simulink model "xsens2kinova"  (R2021a)
settings: Solver=FixedStepAuto  StartTime=0.0  StopTime=inf  FixedStep=0.01  RelTol=1e-3
model workspace (MAT data in the model file):
  MAF_len = 80
undefined symbols (not defined in the file): Attitude, Position, VelocityAtt, VelocityPos
libraries: robotlib x7, dspstat3 x6
settings Model: Creator=user  LastModifiedBy=ywchang
settings SolverCC: AlgebraicLoopSolver=TrustRegion
settings OptimizationCC: EnhancedBackFolding=on  PassReuseOutputArgsAs=Individual arguments  ZeroExternalMemoryAtStartup=off  ZeroInternalMemoryAtStartup=off  MaxStackSize=64  OptimizeBlockOrder=speed  DifferentSizesBufferReuse=on  OptimizationCustomize=off  EfficientTunableParamExpr=on
settings DebuggingCC: ParameterTunabilityLossMsg=error  SFMachineParentedDataDiag=warning
settings HardwareCC: ProdBitPerPointer=32  ProdBitPerSizeT=32  ProdBitPerPtrDiffT=32  ProdLargestAtomicFloat=None  ProdIntDivRoundTo=Undefined  ProdEndianess=Unspecified  ProdWordSize=32  ProdHWDeviceType=Generic->Unspecified (assume 32-bit Generic)  UseEmbeddedCoderFeatures=off
settings SFSimCC: MATLABDynamicMemAlloc=off
settings RTWCC: SystemTargetFile=ert.tlc  HardwareBoard=Robot Operating System (ROS)  TLCOptions="-aInlineSetEventsForThisBaseRateFcn=TLC_FALSE -aSuppressMultiTaskScheduler=TLC_FALSE  -aRateBasedStepFcn=0"  TemplateMakefile=ert_default_tmf  Toolchain=Catkin  TargetLang=C++
settings CodeAppCC: ForceParamTrailComments=on  IgnoreCustomStorageClasses=off  OperatorAnnotations=on  SimulinkDataObjDesc=on  SFDataObjDesc=on  InsertBlockDesc=on
settings ERTTargetCC: SupportNonInlinedSFcns=on

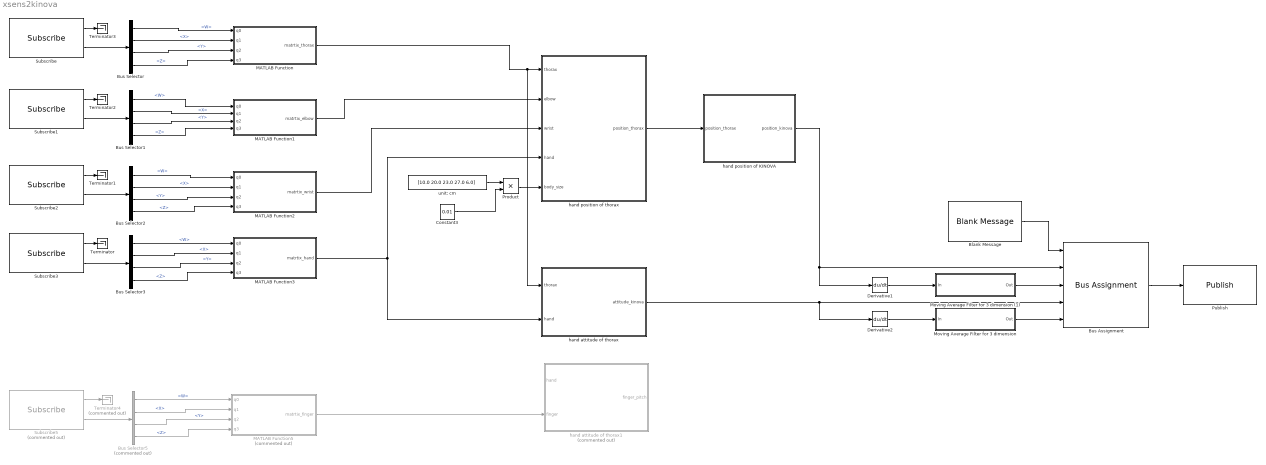
== system xsens2kinova ==
  Blank Message : robotlib/Blank Message  messageClass=Message  entityType=xsens_mtw_driver/xsens2kinova  messageType=xsens_mtw_driver/xsens2kinova  SampleTime=inf  legacyBusStruct=off
  Bus Assignment : BusAssignment  AssignedSignals=Position,VelocityPos,Attitude,VelocityAtt
  Bus Selector{,1..3} (4 alike) : BusSelector  OutputSignals=Orientation.W,Orientation.X,Orientation.Y,Orientation.Z
  Bus Selector5 : BusSelector  Commented=on  OutputSignals=Orientation.W,Orientation.X,Orientation.Y,Orientation.Z
  Constant3 : Constant  Value=0.01
  Derivative1 : Derivative
  Derivative2 : Derivative
  MATLAB Function : MATLAB Function  TreatAsAtomicUnit=on
  MATLAB Function1 : MATLAB Function  TreatAsAtomicUnit=on
  MATLAB Function2 : MATLAB Function  TreatAsAtomicUnit=on
  MATLAB Function3 : MATLAB Function  TreatAsAtomicUnit=on
  MATLAB Function5 : MATLAB Function  Commented=on  TreatAsAtomicUnit=on
  Moving Average Filter for 3 dimension : Subsystem
  Moving Average Filter for 3 dimension (1) : Subsystem
  Product : Product
  Publish : robotlib/Publish  topicSource=Specify your own  topic=/xsens2kinova  messageType=xsens_mtw_driver/xsens2kinova  legacyBusStruct=off  messageQueueLength=1
  Subscribe : robotlib/Subscribe  topicSource=Select from ROS network  topic=/imu_00B47ADF  messageType=sensor_msgs/Imu  SampleTime=-1  legacyBusStruct=off  messageQueueLength=1
  Subscribe1 : robotlib/Subscribe  topicSource=Select from ROS network  topic=/imu_00B47AE4  messageType=sensor_msgs/Imu  SampleTime=-1  legacyBusStruct=off  messageQueueLength=1
  Subscribe2 : robotlib/Subscribe  topicSource=Select from ROS network  topic=/imu_00B47ACF  messageType=sensor_msgs/Imu  SampleTime=-1  legacyBusStruct=off  messageQueueLength=1
  Subscribe3 : robotlib/Subscribe  topicSource=Select from ROS network  topic=/imu_00B47EC3  messageType=sensor_msgs/Imu  SampleTime=-1  legacyBusStruct=off  messageQueueLength=1
  Subscribe5 : robotlib/Subscribe  Commented=on  topicSource=Select from ROS network  topic=/imu_00B47EC4  messageType=sensor_msgs/Imu  SampleTime=-1  legacyBusStruct=off  messageQueueLength=1
  Terminator{,1..3} (4 alike) : Terminator
  Terminator4 : Terminator  Commented=on
  hand attitude of thorax : MATLAB Function  TreatAsAtomicUnit=on
  hand attitude of thorax1 : MATLAB Function  Commented=on  TreatAsAtomicUnit=on
  hand position of KINOVA : MATLAB Function  TreatAsAtomicUnit=on
  hand position of thorax : MATLAB Function  TreatAsAtomicUnit=on
  unit: cm : Constant  Value=[10.0 20.0 23.0 27.0 6.0]
  wires:
  Subscribe/2 -> Bus Selector/1
  Subscribe1/2 -> Bus Selector1/1
  Subscribe2/2 -> Bus Selector2/1
  Subscribe3/2 -> Bus Selector3/1
  MATLAB Function1/1(matrtix_elbow) -> hand position of thorax/2(elbow)
  MATLAB Function2/1(matrtix_wrist) -> hand position of thorax/3(wrist)
  Subscribe5/2 -> Bus Selector5/1
  Bus Selector5/1 -> MATLAB Function5/1(q0)  "<W>"
  Bus Selector5/2 -> MATLAB Function5/2(q1)  "<X>"
  Bus Selector5/3 -> MATLAB Function5/3(q2)  "<Y>"
  Bus Selector5/4 -> MATLAB Function5/4(q3)  "<Z>"
  MATLAB Function3/1(matrtix_hand) -> hand attitude of thorax/2(hand), hand position of thorax/4(hand)
  unit: cm/1 -> Product/1
  Constant3/1 -> Product/2
  Product/1 -> hand position of thorax/5(body_size)
  MATLAB Function/1(matrtix_thorax) -> hand position of thorax/1(thorax), hand attitude of thorax/1(thorax)
  hand position of thorax/1(position_thorax) -> hand position of KINOVA/1(position_thorax)
  hand position of KINOVA/1(position_kinova) -> Bus Assignment/2, Derivative1/1
  Bus Assignment/1 -> Publish/1
  Bus Selector1/3 -> MATLAB Function1/3(q2)  "<Y>"
  Bus Selector/3 -> MATLAB Function/3(q2)  "<Y>"
  Bus Selector/4 -> MATLAB Function/4(q3)  "<Z>"
  Bus Selector/2 -> MATLAB Function/2(q1)  "<X>"
  Bus Selector/1 -> MATLAB Function/1(q0)  "<W>"
  Bus Selector1/4 -> MATLAB Function1/4(q3)  "<Z>"
  Bus Selector1/2 -> MATLAB Function1/2(q1)  "<X>"
  Bus Selector1/1 -> MATLAB Function1/1(q0)  "<W>"
  Bus Selector2/3 -> MATLAB Function2/3(q2)  "<Y>"
  Bus Selector2/2 -> MATLAB Function2/2(q1)  "<X>"
  Bus Selector2/4 -> MATLAB Function2/4(q3)  "<Z>"
  Bus Selector2/1 -> MATLAB Function2/1(q0)  "<W>"
  Bus Selector3/3 -> MATLAB Function3/3(q2)  "<Y>"
  Bus Selector3/4 -> MATLAB Function3/4(q3)  "<Z>"
  Bus Selector3/2 -> MATLAB Function3/2(q1)  "<X>"
  Bus Selector3/1 -> MATLAB Function3/1(q0)  "<W>"
  Subscribe3/1 -> Terminator/1
  Subscribe2/1 -> Terminator1/1
  Subscribe1/1 -> Terminator2/1
  Subscribe/1 -> Terminator3/1
  Subscribe5/1 -> Terminator4/1
  Blank Message/1 -> Bus Assignment/1
  hand attitude of thorax/1(attitude_kinova) -> Derivative2/1, Bus Assignment/4
  MATLAB Function5/1(matrtix_finger) -> hand attitude of thorax1/2(finger)
  Moving Average Filter for 3 dimension/1(Out) -> Bus Assignment/5
  Derivative2/1 -> Moving Average Filter for 3 dimension/1(In)
  Derivative1/1 -> Moving Average Filter for 3 dimension (1)/1(In)
  Moving Average Filter for 3 dimension (1)/1(Out) -> Bus Assignment/3

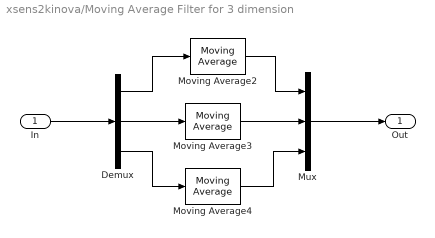
== system xsens2kinova/Moving Average Filter for 3 dimension ==
  In : Inport
  Demux : Demux  Outputs=3
  Moving Average2 : dspstat3/Moving Average  Method=Sliding window  ForgettingFactorPort=off  SpecifyWindowLength=on  WindowLength=MAF_len  ForgettingFactor=0.9  SimulateUsing=Code generation
  Moving Average3 : dspstat3/Moving Average  Method=Sliding window  ForgettingFactorPort=off  SpecifyWindowLength=on  WindowLength=MAF_len  ForgettingFactor=0.9  SimulateUsing=Code generation
  Moving Average4 : dspstat3/Moving Average  Method=Sliding window  ForgettingFactorPort=off  SpecifyWindowLength=on  WindowLength=MAF_len  ForgettingFactor=0.9  SimulateUsing=Code generation
  Mux : Mux  Inputs=3
  Out : Outport
  wires:
  Moving Average3/1 -> Mux/2
  Moving Average4/1 -> Mux/3
  Demux/2 -> Moving Average3/1
  Demux/3 -> Moving Average4/1
  In/1 -> Demux/1
  Moving Average2/1 -> Mux/1
  Demux/1 -> Moving Average2/1
  Mux/1 -> Out/1

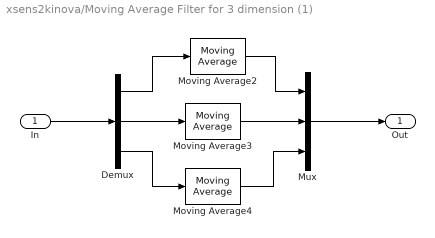
== system xsens2kinova/Moving Average Filter for 3 dimension (1) ==
  In : Inport
  Demux : Demux  Outputs=3
  Moving Average2 : dspstat3/Moving Average  Method=Sliding window  ForgettingFactorPort=off  SpecifyWindowLength=on  WindowLength=MAF_len  ForgettingFactor=0.9  SimulateUsing=Code generation
  Moving Average3 : dspstat3/Moving Average  Method=Sliding window  ForgettingFactorPort=off  SpecifyWindowLength=on  WindowLength=MAF_len  ForgettingFactor=0.9  SimulateUsing=Code generation
  Moving Average4 : dspstat3/Moving Average  Method=Sliding window  ForgettingFactorPort=off  SpecifyWindowLength=on  WindowLength=MAF_len  ForgettingFactor=0.9  SimulateUsing=Code generation
  Mux : Mux  Inputs=3
  Out : Outport
  wires:
  Mux/1 -> Out/1
  Demux/1 -> Moving Average2/1
  Moving Average2/1 -> Mux/1
  In/1 -> Demux/1
  Demux/3 -> Moving Average4/1
  Demux/2 -> Moving Average3/1
  Moving Average4/1 -> Mux/3
  Moving Average3/1 -> Mux/2

== matlab function xsens2kinova/MATLAB Function1 ==
  data: q0 input; matrtix_elbow output; q1 input; q2 input; q3 input
function matrtix_elbow = fcn(q0,q1,q2,q3)



matrtix_elbow=[2*(q0^2+q1^2)-1  2*q1*q2-2*q0*q3  2*q1*q3+2*q0*q2;...
                 2*q1*q2+2*q0*q3  2*(q0^2+q2^2)-1  2*q2*q3-2*q0*q1; ...
                 2*q1*q3-2*q0*q2  2*q2*q3+2*q0*q1  2*(q0^2+q3^2)-1];

== matlab function xsens2kinova/MATLAB Function ==
  data: q0 input; matrtix_thorax output; q1 input; q2 input; q3 input
function matrtix_thorax = fcn(q0,q1,q2,q3)

% q1=-q1;
% q2=-q2;
% q3=-q3;

matrtix_thorax=[2*(q0^2+q1^2)-1  2*q1*q2-2*q0*q3  2*q1*q3+2*q0*q2;...
                 2*q1*q2+2*q0*q3  2*(q0^2+q2^2)-1  2*q2*q3-2*q0*q1; ...
                 2*q1*q3-2*q0*q2  2*q2*q3+2*q0*q1  2*(q0^2+q3^2)-1];

== matlab function xsens2kinova/MATLAB Function2 ==
  data: q0 input; matrtix_wrist output; q1 input; q2 input; q3 input
function matrtix_wrist = fcn(q0,q1,q2,q3)



matrtix_wrist=[2*(q0^2+q1^2)-1  2*q1*q2-2*q0*q3  2*q1*q3+2*q0*q2;...
                 2*q1*q2+2*q0*q3  2*(q0^2+q2^2)-1  2*q2*q3-2*q0*q1; ...
                 2*q1*q3-2*q0*q2  2*q2*q3+2*q0*q1  2*(q0^2+q3^2)-1];

== matlab function xsens2kinova/MATLAB Function3 ==
  data: q0 input; matrtix_hand output; q1 input; q2 input; q3 input
function matrtix_hand = fcn(q0,q1,q2,q3)



matrtix_hand=[2*(q0^2+q1^2)-1  2*q1*q2-2*q0*q3  2*q1*q3+2*q0*q2;...
                 2*q1*q2+2*q0*q3  2*(q0^2+q2^2)-1  2*q2*q3-2*q0*q1; ...
                 2*q1*q3-2*q0*q2  2*q2*q3+2*q0*q1  2*(q0^2+q3^2)-1];

== matlab function xsens2kinova/hand position of thorax ==
  data: thorax input; position_thorax output; elbow input; wrist input; hand input; body_size input
function position_thorax = fcn(thorax, elbow, wrist, hand, body_size)

thorax=thorax^-1;
shoulder_position = [-body_size(1) -body_size(2) 0]';
upperarm_position = thorax*(elbow*[body_size(3) 0 0]');
forearm_position = thorax*(wrist*[body_size(4) 0 0]');
hand_position = thorax*(hand*[body_size(5) 0 0]');

position_thorax = shoulder_position + upperarm_position + forearm_position + hand_position;

== matlab function xsens2kinova/hand position of KINOVA ==
  data: position_thorax input; position_kinova output
function position_kinova = fcn(position_thorax)

thorax_to_kinova_base=[0 0 1;0 1 0;-1 0 0];
position_kinova = thorax_to_kinova_base*position_thorax;

== matlab function xsens2kinova/hand attitude of thorax ==
  data: thorax input; attitude_kinova output; hand input
function attitude_kinova = fcn(thorax, hand)

thorax = thorax^-1;
thorax_to_kinova_base=[0 0 1;0 1 0;-1 0 0];

% 加入軸角表示式
A = thorax_to_kinova_base*thorax*hand;
theta0e = rotm2axang(A).';
attitude_kinova = theta0e(1:3)*theta0e(4); % axis angle

== matlab function xsens2kinova/MATLAB Function5 ==
  data: q0 input; matrtix_finger output; q1 input; q2 input; q3 input
function matrtix_finger = fcn(q0,q1,q2,q3)

matrtix_finger=[2*(q0^2+q1^2)-1  2*q1*q2-2*q0*q3  2*q1*q3+2*q0*q2;...
                 2*q1*q2+2*q0*q3  2*(q0^2+q2^2)-1  2*q2*q3-2*q0*q1; ...
                 2*q1*q3-2*q0*q2  2*q2*q3+2*q0*q1  2*(q0^2+q3^2)-1];

== matlab function xsens2kinova/hand attitude of thorax1 ==
  data: hand input; finger input; finger_pitch output
function finger_pitch = fcn(hand, finger)

hand = hand^-1;
Rhf = hand*finger;
finger_pitch = -asin(Rhf(3,1));
